simulink model "Differential_MP_TS9"  (Simulink 7.6)
settings: Solver=ode45  SolverMode=SingleTasking  StartTime=0  StopTime=25  FixedStep=0.002  RelTol=1e-3  AbsTol=1e-6
libraries: Solver_SF x1
settings Model: Creator=pmather  LastModifiedBy=mkhan  ExtModeTrigMode=oneshot  ExtModeArmWhenConnect=off
settings DataIOCC: LimitDataPoints=off  SignalLoggingName=sigsOut
settings OptimizationCC: BlockReduction=off  BooleanDataType=off
settings DebuggingCC: SaveWithParameterizedLinksMsg=none  SignalResolutionControl=TryResolveAllWithWarning  SolverPrmCheckMsg=none  MultiTaskDSMMsg=warning  MultiTaskCondExecSysMsg=none  StrictBusMsg=None
settings HardwareCC: TargetUnknown=on
settings RTWCC: TemplateMakefile=grt_vc.tmf  IncludeERTFirstTime=on
settings GRTTargetCC: TargetFcnLib=ansi_tfl_tmw.mat

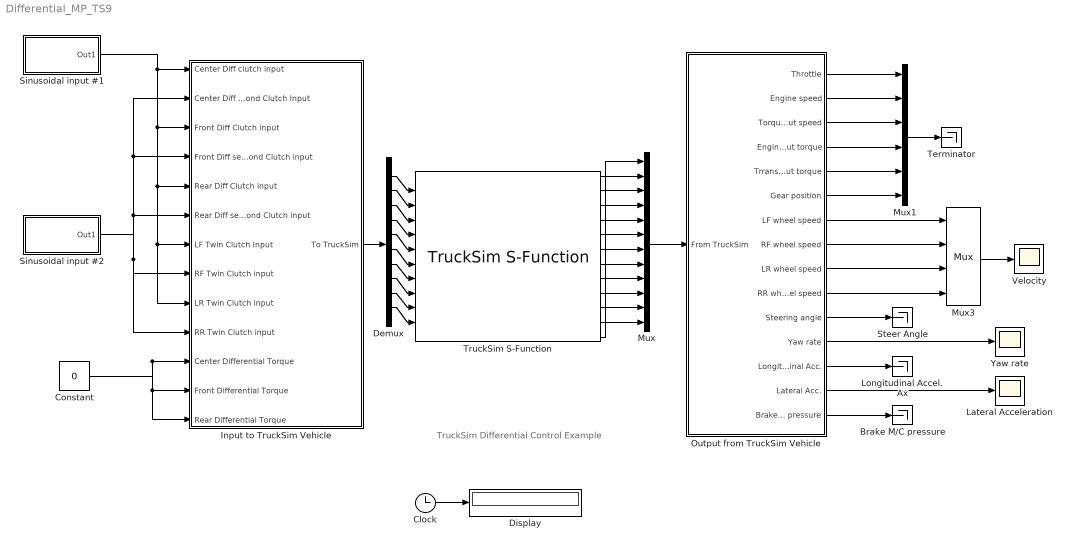
== system Differential_MP_TS9 ==
  note: TruckSim Differential Control Example
  Brake M/C pressure : Terminator
  Clock : Clock
      settings: Decimation=10
  Constant : Constant  Value=0
  Demux : Demux  Outputs=10
  Display : Display
      settings: Format=bank  Decimation=100
  Input to TruckSim Vehicle : Subsystem
  Lateral Acceleration : Scope
      settings: TickLabels=on  YMin=-0.2  YMax=0.2  DataFormat=Array  SampleTime=100
  Longitudinal Accel. Ax : Terminator
  Mux : Mux  Inputs=12
  Mux1 : Mux  Inputs=6
  Mux3 : Mux
  Output from TruckSim Vehicle : Subsystem
  Sinusoidal input #1 : Subsystem
  Sinusoidal input #2 : Subsystem
  Steer Angle : Terminator
  Terminator : Terminator
  TruckSim S-Function : Solver_SF/TruckSim S-Function  Priority=1  SIMFILE=simfile.sim
  Velocity : Scope
      settings: TickLabels=on  YMin=-20  YMax=100  DataFormat=Array  SampleTime=100
  Yaw rate : Scope
      settings: TickLabels=on  DataFormat=Array  SampleTime=100
  wires:
  Sinusoidal input #1/1(Out1) -> Input to TruckSim Vehicle/1(Center Diff clutch input), Input to TruckSim Vehicle/3(Front Diff Clutch input), Input to TruckSim Vehicle/5(Rear Diff Clutch input), Input to TruckSim Vehicle/7(LF Twin Clutch Input), Input to TruckSim Vehicle/9(LR Twin Clutch input)
  Constant/1 -> Input to TruckSim Vehicle/11(Center Differential Torque), Input to TruckSim Vehicle/12("Front Differential Torque "), Input to TruckSim Vehicle/13(Rear Differential Torque)
  Mux3/1 -> Velocity/1
  Output from TruckSim Vehicle/7(LF wheel speed) -> Mux3/1
  Output from TruckSim Vehicle/8(RF wheel speed) -> Mux3/2
  Output from TruckSim Vehicle/9(LR wheel speed) -> Mux3/3
  Output from TruckSim Vehicle/10(RR wheel speed) -> Mux3/4
  Output from TruckSim Vehicle/12(Yaw rate) -> Yaw rate/1
  Output from TruckSim Vehicle/14(Lateral Acc.) -> Lateral Acceleration/1
  Output from TruckSim Vehicle/11(Steering angle) -> Steer Angle/1
  Output from TruckSim Vehicle/13(Longitudinal Acc.) -> Longitudinal Accel. Ax/1
  Output from TruckSim Vehicle/15(Brake M/C pressure) -> Brake M/C pressure/1
  Sinusoidal input #2/1(Out1) -> Input to TruckSim Vehicle/8(RF Twin Clutch input), Input to TruckSim Vehicle/6(Rear Diff second Clutch input), Input to TruckSim Vehicle/4(Front Diff second Clutch input), Input to TruckSim Vehicle/2(Center Diff second Clutch Input), Input to TruckSim Vehicle/10(RR Twin Clutch input)
  Clock/1 -> Display/1
  Mux/1 -> Output from TruckSim Vehicle/1(From TruckSim)
  TruckSim S-Function/1 -> Mux/1
  TruckSim S-Function/12 -> Mux/12
  TruckSim S-Function/11 -> Mux/11
  TruckSim S-Function/10 -> Mux/10
  TruckSim S-Function/9 -> Mux/9
  TruckSim S-Function/8 -> Mux/8
  TruckSim S-Function/7 -> Mux/7
  TruckSim S-Function/6 -> Mux/6
  TruckSim S-Function/5 -> Mux/5
  TruckSim S-Function/4 -> Mux/4
  TruckSim S-Function/3 -> Mux/3
  TruckSim S-Function/2 -> Mux/2
  Mux1/1 -> Terminator/1
  Output from TruckSim Vehicle/1(Throttle) -> Mux1/1
  Output from TruckSim Vehicle/6(Gear position) -> Mux1/6
  Output from TruckSim Vehicle/2(Engine speed) -> Mux1/2
  Output from TruckSim Vehicle/3(Torque converter output speed) -> Mux1/3
  Output from TruckSim Vehicle/4(Engine output torque) -> Mux1/4
  Output from TruckSim Vehicle/5(Trransmission output torque) -> Mux1/5
  Demux/1 -> TruckSim S-Function/1
  Demux/10 -> TruckSim S-Function/10
  Demux/9 -> TruckSim S-Function/9
  Demux/8 -> TruckSim S-Function/8
  Demux/7 -> TruckSim S-Function/7
  Demux/6 -> TruckSim S-Function/6
  Demux/5 -> TruckSim S-Function/5
  Demux/3 -> TruckSim S-Function/3
  Demux/2 -> TruckSim S-Function/2
  Demux/4 -> TruckSim S-Function/4
  Input to TruckSim Vehicle/1(To TruckSim) -> Demux/1

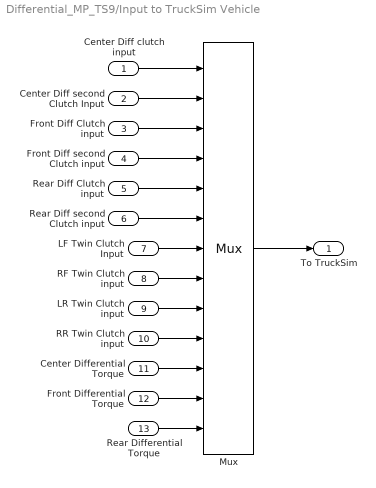
== system Differential_MP_TS9/Input to TruckSim Vehicle ==
  Center Diff clutch input : Inport
  Center Diff second Clutch Input : Inport  Port=2
  Front Diff Clutch input : Inport  Port=3
  Front Diff second Clutch input : Inport  Port=4
  Rear Diff Clutch input : Inport  Port=5
  Rear Diff second Clutch input : Inport  Port=6
  LF Twin Clutch Input : Inport  Port=7
  RF Twin Clutch input : Inport  Port=8
  LR Twin Clutch input : Inport  Port=9
  RR Twin Clutch input : Inport  Port=10
  Center Differential Torque : Inport  Port=11
  "Front Differential Torque " : Inport  Port=12
  Rear Differential Torque : Inport  Port=13
  Mux : Mux  Inputs=13
  To TruckSim : Outport
  wires:
  Mux/1 -> To TruckSim/1
  Center Differential Torque/1 -> Mux/11
  Rear Differential Torque/1 -> Mux/13
  "Front Differential Torque "/1 -> Mux/12
  RR Twin Clutch input/1 -> Mux/10
  LR Twin Clutch input/1 -> Mux/9
  RF Twin Clutch input/1 -> Mux/8
  LF Twin Clutch Input/1 -> Mux/7
  Rear Diff second Clutch input/1 -> Mux/6
  Rear Diff Clutch input/1 -> Mux/5
  Front Diff second Clutch input/1 -> Mux/4
  Front Diff Clutch input/1 -> Mux/3
  Center Diff second Clutch Input/1 -> Mux/2
  Center Diff clutch input/1 -> Mux/1

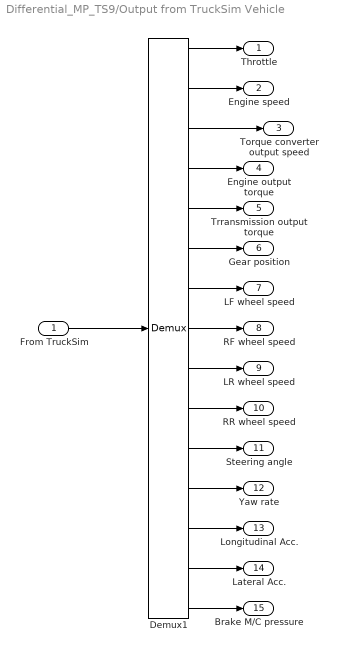
== system Differential_MP_TS9/Output from TruckSim Vehicle ==
  From TruckSim : Inport
  Demux1 : Demux  Outputs=15
  Throttle : Outport
  Engine speed : Outport  Port=2
  Torque converter output speed : Outport  Port=3
  Engine output torque : Outport  Port=4
  Trransmission output torque : Outport  Port=5
  Gear position : Outport  Port=6
  LF wheel speed : Outport  Port=7
  RF wheel speed : Outport  Port=8
  LR wheel speed : Outport  Port=9
  RR wheel speed : Outport  Port=10
  Steering angle : Outport  Port=11
  Yaw rate : Outport  Port=12
  Longitudinal Acc. : Outport  Port=13
  Lateral Acc. : Outport  Port=14
  Brake M/C pressure : Outport  Port=15
  wires:
  From TruckSim/1 -> Demux1/1
  Demux1/1 -> Throttle/1
  Demux1/2 -> Engine speed/1
  Demux1/3 -> Torque converter output speed/1
  Demux1/7 -> LF wheel speed/1
  Demux1/13 -> Longitudinal Acc./1
  Demux1/14 -> Lateral Acc./1
  Demux1/15 -> Brake M/C pressure/1
  Demux1/8 -> RF wheel speed/1
  Demux1/9 -> LR wheel speed/1
  Demux1/10 -> RR wheel speed/1
  Demux1/11 -> Steering angle/1
  Demux1/12 -> Yaw rate/1
  Demux1/4 -> Engine output torque/1
  Demux1/5 -> Trransmission output torque/1
  Demux1/6 -> Gear position/1

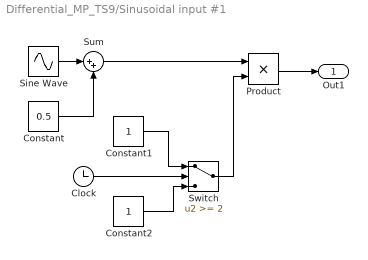
== system Differential_MP_TS9/Sinusoidal input #1 ==
  Clock : Clock
      settings: Decimation=10
  Constant : Constant  Value=0.5
  Constant1 : Constant
  Constant2 : Constant
  Product : Product  SaturateOnIntegerOverflow=on  InputSameDT=on  OutDataTypeStr=Inherit: Same as first input
  Sine Wave : Sin  Amplitude=0.5  Frequency=0.25*2*pi  Phase=3/2*pi
  Sum : Sum  Inputs=|++  SaturateOnIntegerOverflow=on  InputSameDT=on  OutDataTypeStr=Inherit: Same as first input
  Switch : Switch  Threshold=2  SaturateOnIntegerOverflow=on  InputSameDT=on
  Out1 : Outport
  wires:
  Sine Wave/1 -> Sum/1
  Constant/1 -> Sum/2
  Clock/1 -> Switch/2
  Constant1/1 -> Switch/1
  Constant2/1 -> Switch/3
  Switch/1 -> Product/2
  Product/1 -> Out1/1
  Sum/1 -> Product/1

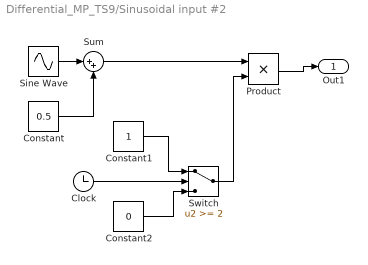
== system Differential_MP_TS9/Sinusoidal input #2 ==
  Clock : Clock
      settings: Decimation=10
  Constant : Constant  Value=0.5
  Constant1 : Constant
  Constant2 : Constant  Value=0
  Product : Product  SaturateOnIntegerOverflow=on  InputSameDT=on  OutDataTypeStr=Inherit: Same as first input
  Sine Wave : Sin  Amplitude=0.5  Frequency=0.25*2*pi  Phase=1/2*pi
  Sum : Sum  Inputs=|++  SaturateOnIntegerOverflow=on  InputSameDT=on  OutDataTypeStr=Inherit: Same as first input
  Switch : Switch  Threshold=2  SaturateOnIntegerOverflow=on  InputSameDT=on
  Out1 : Outport
  wires:
  Sine Wave/1 -> Sum/1
  Constant/1 -> Sum/2
  Clock/1 -> Switch/2
  Constant1/1 -> Switch/1
  Constant2/1 -> Switch/3
  Switch/1 -> Product/2
  Product/1 -> Out1/1
  Sum/1 -> Product/1
